simulink model "li_slotine"  (R2020b)
settings: Solver=VariableStepAuto  StartTime=0.0  StopTime=time  RelTol=1e-3
values from neighbouring files (symbols this model uses):
  Ath = 0.5    [main.m]
  b = sym('b','real')    [Oss_par.m]    (also in main.m = 0.2)
  gravity = sym('gravity','real')    [Oss_par.m]    (also in main.m = 9.81)
  I = sym('I','real')    [Oss_par.m]    (also in main.m = 235.2)
  K = sym('K','real')    [Oss_par.m]    (also in main.m = 40.248)
  L = sym('L','real')    [Oss_par.m]    (also in dir_der.m = h * f; main.m = 2.1)
  lambda = 5    [main.m]
  m = sym('m','real')    [Oss_par.m]    (also in main.m = 160)
  R = sym('R','real')    [Oss_par.m]    (also in main.m = 0.6)
  selector = select(1)    [main.m]    (also in select.m = input('? '))
  wth = 0.2    [main.m]
settings Model: Creator=Tommaso  LastModifiedBy=Tommaso
settings DataIOCC: ReturnWorkspaceOutputs=off

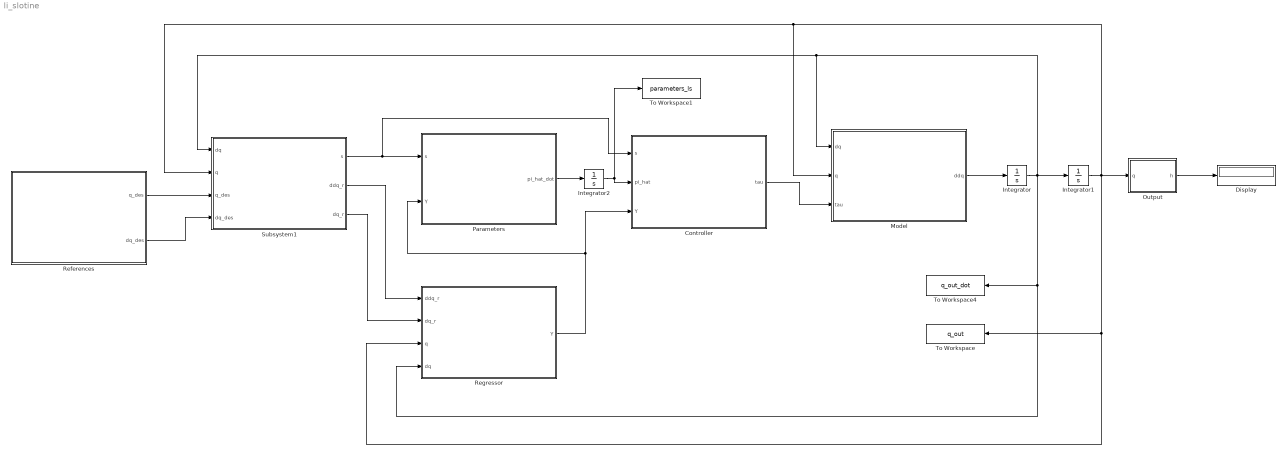
== system li_slotine ==
  Controller : MATLAB Function  TreatAsAtomicUnit=on
  Display : Display
  Integrator : Integrator  InitialCondition=[0; 0]
  Integrator1 : Integrator  InitialCondition=[0; pi/12]
  Integrator2 : Integrator  InitialCondition=[0; 0; 0; 0]
  Model : MATLAB Function  TreatAsAtomicUnit=on
  Output : MATLAB Function  TreatAsAtomicUnit=on
  Parameters : MATLAB Function  TreatAsAtomicUnit=on
  References : Subsystem
  Regressor : MATLAB Function  TreatAsAtomicUnit=on
  Subsystem1 : Subsystem
  To Workspace : ToWorkspace  VariableName=q_out  SaveFormat=Timeseries  SampleTime=-1
  To Workspace1 : ToWorkspace  VariableName=parameters_ls  SaveFormat=Timeseries  SampleTime=-1
  To Workspace4 : ToWorkspace  VariableName=q_out_dot  SaveFormat=Timeseries  SampleTime=-1
  wires:
  Model/1(ddq) -> Integrator/1
  Controller/1(tau) -> Model/3(tau)
  Parameters/1(pi_hat_dot) -> Integrator2/1
  Output/1(h) -> Display/1
  Integrator1/1 -> Regressor/3(q), To Workspace/1, Output/1(q), Model/2(q), Subsystem1/2(q)
  Integrator/1 -> Integrator1/1, Subsystem1/1(dq), Model/1(dq), Regressor/4(dq), To Workspace4/1
  Integrator2/1 -> To Workspace1/1, Controller/2(pi_hat)
  Regressor/1(Y) -> Controller/3(Y), Parameters/2(Y)
  Subsystem1/1(s) -> Controller/1(s), Parameters/1(s)
  Subsystem1/2(ddq_r) -> Regressor/1(ddq_r)
  Subsystem1/3(dq_r) -> Regressor/2(dq_r)
  References/1(q_des) -> Subsystem1/3(q_des)
  References/2(dq_des) -> Subsystem1/4(dq_des)

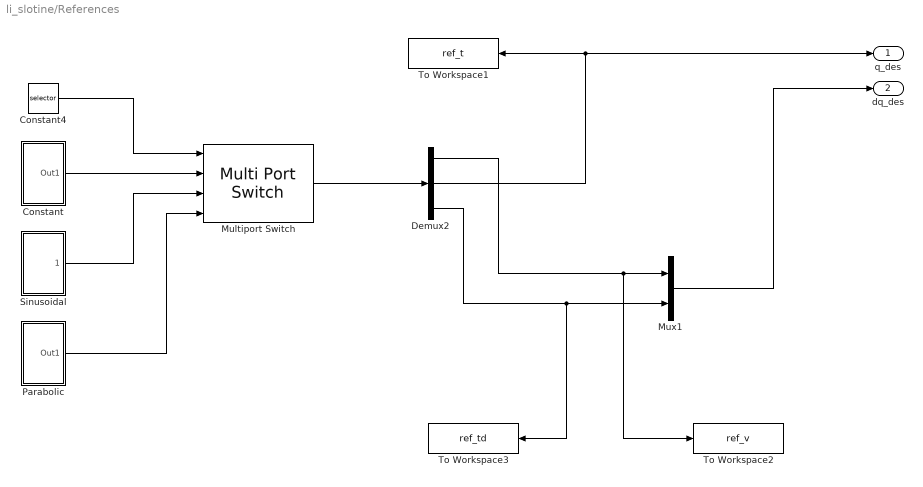
== system li_slotine/References ==
  Constant : Subsystem
  Constant4 : Constant  Value=selector
  Demux2 : Demux  Outputs=3
  Multiport Switch : MultiPortSwitch
  Mux1 : Mux  Inputs=2
  Parabolic : Subsystem
  Sinusoidal : Subsystem
  To Workspace1 : ToWorkspace  VariableName=ref_t  SaveFormat=Timeseries  SampleTime=-1
  To Workspace2 : ToWorkspace  VariableName=ref_v  SaveFormat=Timeseries  SampleTime=-1
  To Workspace3 : ToWorkspace  VariableName=ref_td  SaveFormat=Timeseries  SampleTime=-1
  q_des : Outport
  dq_des : Outport  Port=2
  wires:
  Mux1/1 -> dq_des/1
  Demux2/2 -> q_des/1, To Workspace1/1
  Multiport Switch/1 -> Demux2/1
  Sinusoidal/1(Outport) -> Multiport Switch/3
  Constant4/1 -> Multiport Switch/1
  Parabolic/1(Out1) -> Multiport Switch/4
  Demux2/1 -> To Workspace2/1, Mux1/1
  Constant/1(Out1) -> Multiport Switch/2
  Demux2/3 -> To Workspace3/1, Mux1/2

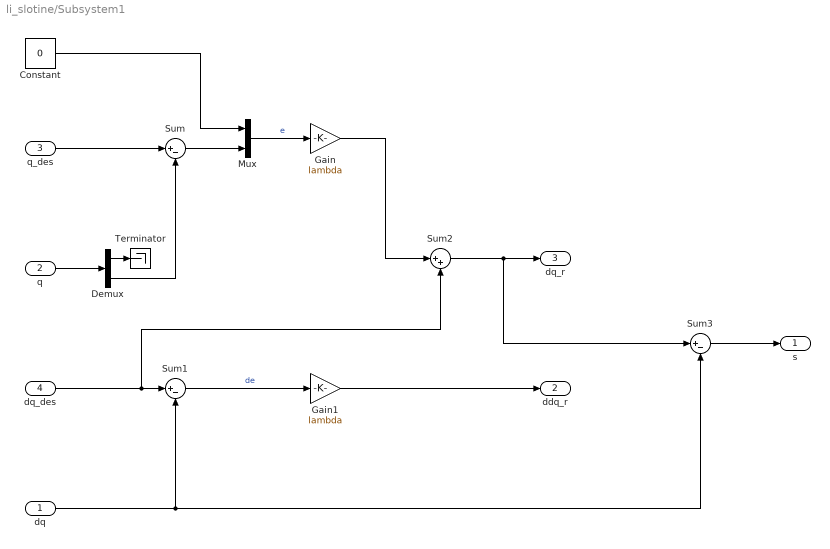
== system li_slotine/Subsystem1 ==
  dq : Inport
  q : Inport  Port=2
  q_des : Inport  Port=3
  dq_des : Inport  Port=4
  Constant : Constant  Value=0
  Demux : Demux  Outputs=2
  Gain : Gain  Gain=lambda
  Gain1 : Gain  Gain=lambda
  Mux : Mux  Inputs=2
  Sum : Sum  Inputs=|+-
  Sum1 : Sum  Inputs=|+-
  Sum2 : Sum  Inputs=|++
  Sum3 : Sum  Inputs=|+-
  Terminator : Terminator
  s : Outport
  ddq_r : Outport  Port=2
  dq_r : Outport  Port=3
  wires:
  q_des/1 -> Sum/1
  q/1 -> Demux/1
  Demux/2 -> Sum/2
  Demux/1 -> Terminator/1
  Sum/1 -> Mux/2
  Constant/1 -> Mux/1
  dq_des/1 -> Sum2/2, Sum1/1
  dq/1 -> Sum3/2, Sum1/2
  Mux/1 -> Gain/1  "e"
  Gain/1 -> Sum2/1
  Sum2/1 -> Sum3/1, dq_r/1
  Sum1/1 -> Gain1/1  "de"
  Gain1/1 -> ddq_r/1
  Sum3/1 -> s/1

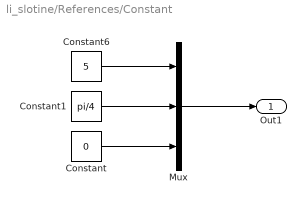
== system li_slotine/References/Constant ==
  Constant : Constant  Value=0
  Constant1 : Constant  Value=pi/4
  Constant6 : Constant  Value=5
  Mux : Mux  Inputs=3
  Out1 : Outport
  wires:
  Constant1/1 -> Mux/2
  Constant/1 -> Mux/3
  Mux/1 -> Out1/1
  Constant6/1 -> Mux/1

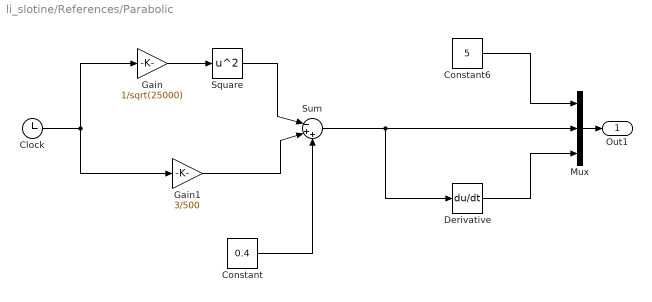
== system li_slotine/References/Parabolic ==
  Clock : Clock
  Constant : Constant  Value=0.4
  Constant6 : Constant  Value=5
  Derivative : Derivative
  Gain : Gain  Gain=1/sqrt(25000)
  Gain1 : Gain  Gain=3/500
  Mux : Mux  Inputs=3
  Square : Math  Operator=square  SaturateOnIntegerOverflow=on
  Sum : Sum  Inputs=|-++
  Out1 : Outport
  wires:
  Mux/1 -> Out1/1
  Gain/1 -> Square/1
  Derivative/1 -> Mux/3
  Square/1 -> Sum/1
  Sum/1 -> Mux/2, Derivative/1
  Gain1/1 -> Sum/2
  Clock/1 -> Gain1/1, Gain/1
  Constant6/1 -> Mux/1
  Constant/1 -> Sum/3

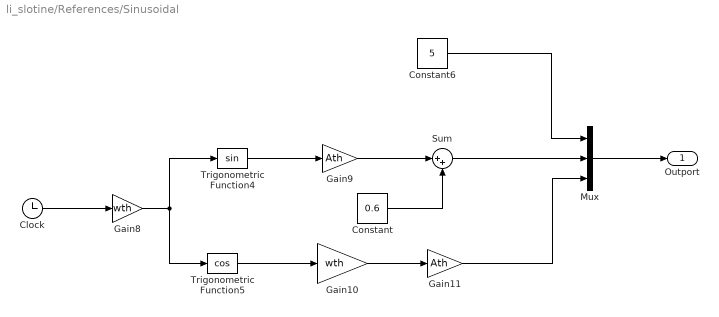
== system li_slotine/References/Sinusoidal ==
  Clock : Clock
  Constant : Constant  Value=0.6
  Constant6 : Constant  Value=5
  Gain10 : Gain  Gain=wth
  Gain11 : Gain  Gain=Ath
  Gain8 : Gain  Gain=wth
  Gain9 : Gain  Gain=Ath
  Mux : Mux  Inputs=3
  Sum : Sum  Inputs=|++
  Trigonometric Function4 : Trigonometry
  Trigonometric Function5 : Trigonometry  Operator=cos
  Outport : Outport
  wires:
  Gain11/1 -> Mux/3
  Trigonometric Function5/1 -> Gain10/1
  Gain10/1 -> Gain11/1
  Gain8/1 -> Trigonometric Function4/1, Trigonometric Function5/1
  Constant/1 -> Sum/2
  Clock/1 -> Gain8/1
  Gain9/1 -> Sum/1
  Mux/1 -> Outport/1
  Trigonometric Function4/1 -> Gain9/1
  Sum/1 -> Mux/2
  Constant6/1 -> Mux/1

== matlab function li_slotine/Output ==
  data: q input; h output; L parameter
function h = output(q, L)

% Output 
h = L*sin(q(2)); % [m]

== matlab function li_slotine/Model ==
  data: m parameter; R parameter; gravity parameter; L parameter; dq input; K parameter; b parameter; I parameter; q input; tau input; ddq output
function ddq = model(m, R, gravity, L, dq, K, b, I, q, tau)

% Configuration variables
theta = q(2);
x_dot = dq(1);

% Inertial matrix (2x2)
M = [m*R 0; 0 I];

% Damping matrix (2x2)
C = [(R/2)*K*(1+sin(theta))*x_dot 0; -(L/4)*K*(1+sin(theta))*x_dot*sin(theta) b];

% Potential vector (2x1)
G = [0; m*gravity*(L/2)*cos(theta)];

% Dynamic equation
ddq = M^(-1)*(tau - C*dq - G);

== matlab function li_slotine/Controller ==
  data: s input; pi_hat input; Y input; tau output size=2; selector parameter
function tau = controller(s, pi_hat, Y, selector)

% Proportional gain 
Kd = 500*eye(2); % 900 per parabola
if selector == 3
    Kd = 900*eye(2);
end
% Control output (2x1)
tau = Y * pi_hat + Kd * s;

== matlab function li_slotine/Parameters ==
  data: s input; pi_hat_dot output; Y input
function pi_hat_dot = pi_hat_dot(s, Y)

% Dynamic parameters derivate (4x1)
pi_hat_dot = Y' * s;

== matlab function li_slotine/Regressor ==
  data: ddq_r input; Y output; dq_r input; q input; dq input; R parameter; gravity parameter; L parameter
function Y = Y_function(ddq_r, dq_r, q, dq, R, gravity, L)

% Configuration variables
theta = q(2);
x_dot = dq(1);
x_dot_r = dq_r(1);
theta_dot_r = dq_r(2);
x_ddot_r = ddq_r(1);
theta_ddot_r = ddq_r(2);

% Dynamic regressor (2x4)
Y = [R*x_ddot_r, 0, 0, R*(x_dot*x_dot_r*(1+sin(theta)))/2; gravity*(L/2)*cos(theta), theta_ddot_r, theta_dot_r, -(L/4)*(x_dot*x_dot_r*sin(theta)*(1+sin(theta)))];
